simulink model "Lab2Skeleton"  (R2022a)
settings: Solver=ode1  StartTime=0.0  StopTime=70  FixedStep=0.01  RelTol=1e-3  EnableMultiTasking=on
PostLoadFcn:
  | p=1:640; % pixels from left to right
  | 
  | Obtained_angles=(320-p).*(57/640)*pi./180;  % Kinect's horizontal FOV = 57 degrees
  | 
  | S=400; % S = Size of the 2D Map matrix... the highet S is the higher resolution we would end up with - %00 might be high for Embedded computing
undefined symbols (not defined in the file): HIL, qc_get_step_size
libraries: quarc_library x4
settings Model: ExtModeTrigDuration=2  Creator=drmadill  LastModifiedBy=jonic
settings SolverCC: AlgebraicLoopSolver=TrustRegion  PositivePriorityOrder=on
settings DataIOCC: SaveOutput=off  SignalLogging=off  DSMLogging=off  SaveTime=off  ReturnWorkspaceOutputs=off
settings DebuggingCC: UnconnectedInputMsg=warning  UnconnectedOutputMsg=warning  UnconnectedLineMsg=warning  SFMachineParentedDataDiag=warning  ArithmeticOperatorsInVariantConditions=warning
settings SFSimCC: SimUseLocalCustomCode=off  CustomCodeUndefinedFunction=UseInterfaceOnly
settings RTWCC: Description=Generic Real-Time Target  RTWUseLocalCustomCode=off
settings CodeAppCC: StateflowObjectComments=on
settings ConfigComp: CovMetricSettings=dswe

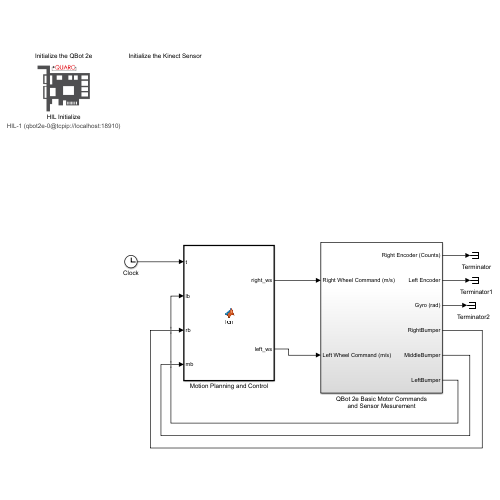
[thumbnail: Simulink's stored preview of the top-level diagram]
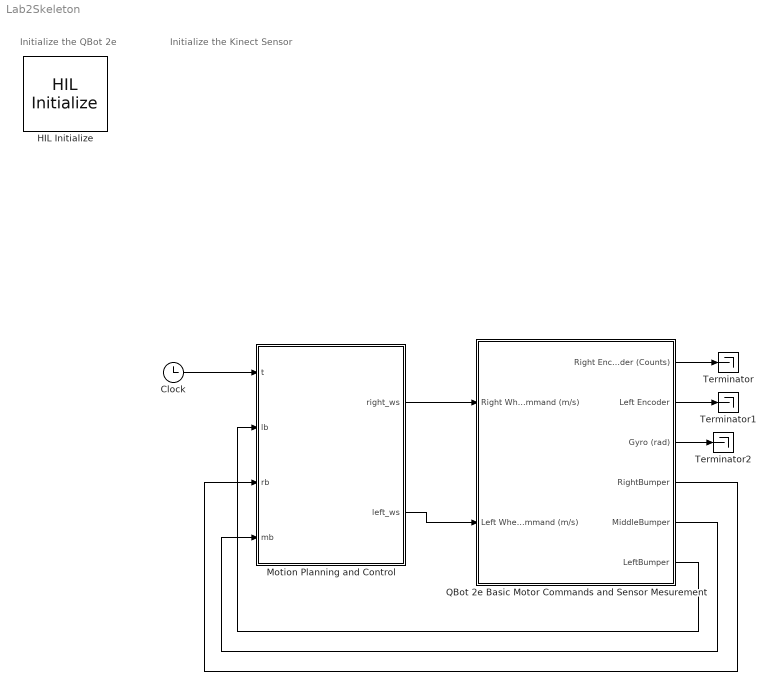
== system Lab2Skeleton ==
  note: Initialize the Kinect Sensor
  note: Initialize the QBot 2e
  Clock : Clock
  HIL Initialize : quarc_library/Data Acquisition/Generic/Configuration/HIL Initialize  Priority=-99  object_name=HIL-1  board_type=qbot2e  board_number=0@tcpip://localhost:18910  board_options=pwm0_en=1;pwm0_pin=12;pwm1_en=1;pwm1_pin=13;  exclusive=off  active=on  hardware_clocks=[]  clock_modes=[]  initial_clock_frequencies=[]  set_clock_params_at_start=off  set_clock_params_at_switch_in=off  set_clock_frequencies_at_start=off  set_clock_frequencies_at_switch_in=off  analog_input_channels=[0:5]  analog_input_configurations=[]  analog_input_maximums=[16.5 3.3 3.3 3.3 3.3 3.3]  analog_input_minimums=[0 0 0 0 0 0]  set_analog_input_params_at_start=off  set_analog_input_params_at_switch_in=off  analog_output_channels=[]  analog_output_maximums=[]  analog_output_minimums=[]  initial_analog_outputs=[]  final_analog_outputs=[]  watchdog_analog_outputs=[]  set_analog_output_params_at_start=off  set_analog_output_params_at_switch_in=off  set_analog_outputs_at_start=off  set_analog_outputs_at_switch_in=off  set_analog_outputs_at_terminate=off  set_analog_outputs_at_switch_out=off  set_analog_outputs_on_watchdog=off  digital_input_channels=[28:58]  digital_output_channels=[28:31]  digital_output_configuration=[]  initial_digital_outputs=[0]  final_digital_outputs=[0]  watchdog_digital_outputs=[]  set_digital_output_params_at_start=off  set_digital_output_params_at_switch_in=off  set_digital_outputs_at_start=on  set_digital_outputs_at_switch_in=off  set_digital_outputs_at_terminate=on  set_digital_outputs_at_switch_out=off  set_digital_outputs_on_watchdog=off  encoder_channels=[0:1]  quadrature=[4]  encoder_filter_frequency=[]  initial_encoder_counts=[0]  set_encoder_params_at_start=on  set_encoder_params_at_switch_in=off  set_encoder_counts_at_start=on  set_encoder_counts_at_switch_in=off  pwm_channels=[0:1]  pwm_modes=0  pwm_frequency=100e6 / 4095  pwm_configuration=[0]  pwm_alignment=[0]  pwm_polarity=[1]  pwm_leading_deadband=[]  pwm_trailing_deadband=[]  initial_pwm_outputs=[0]  final_pwm_outputs=[0]  watchdog_pwm_outputs=[]  set_pwm_params_at_start=on  set_pwm_params_at_switch_in=off  set_pwm_outputs_at_start=on  set_pwm_outputs_at_switch_in=off  set_pwm_outputs_at_terminate=on  set_pwm_outputs_at_switch_out=off  set_pwm_outputs_on_watchdog=off  other_output_channels=[2000:2001 14000 16000]  initial_other_outputs=[0 0 0 7]  final_other_outputs=[0 0 0 7]  watchdog_other_outputs=[]  set_other_outputs_at_start=on  set_other_outputs_at_switch_in=off  set_other_outputs_at_terminate=on  set_other_outputs_at_switch_out=off  set_other_outputs_on_watchdog=off
  Motion Planning and Control : MATLAB Function  TreatAsAtomicUnit=on  SystemSampleTime=qc_get_step_size
  QBot 2e Basic Motor Commands and Sensor Mesurement : Subsystem
  Terminator : Terminator
  Terminator1 : Terminator
  Terminator2 : Terminator
  wires:
  Clock/1 -> Motion Planning and Control/1(t)
  QBot 2e Basic Motor Commands and Sensor Mesurement/4(RightBumper) -> Motion Planning and Control/3(rb)
  QBot 2e Basic Motor Commands and Sensor Mesurement/5(MiddleBumper) -> Motion Planning and Control/4(mb)
  QBot 2e Basic Motor Commands and Sensor Mesurement/6(LeftBumper) -> Motion Planning and Control/2(lb)
  Motion Planning and Control/1(right_ws) -> QBot 2e Basic Motor Commands and Sensor Mesurement/1(Right Wheel Command (m/s))
  Motion Planning and Control/2(left_ws) -> QBot 2e Basic Motor Commands and Sensor Mesurement/2(Left Wheel Command (m/s))
  QBot 2e Basic Motor Commands and Sensor Mesurement/1(Right Encoder (Counts)) -> Terminator/1
  QBot 2e Basic Motor Commands and Sensor Mesurement/2(Left Encoder) -> Terminator1/1
  QBot 2e Basic Motor Commands and Sensor Mesurement/3(Gyro (rad)) -> Terminator2/1

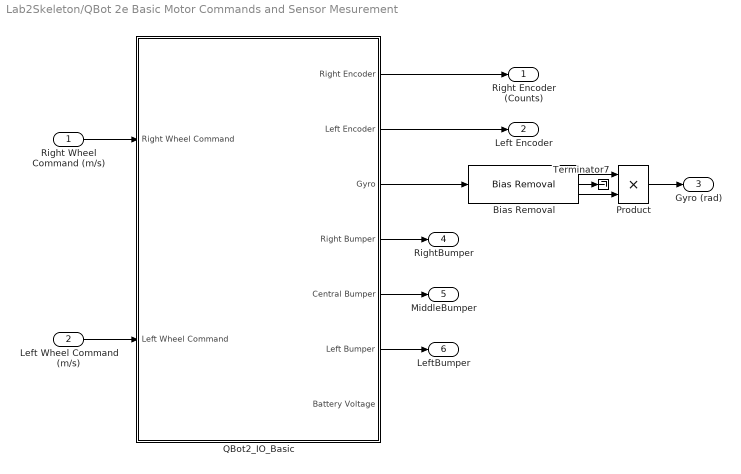
== system Lab2Skeleton/QBot 2e Basic Motor Commands and Sensor Mesurement ==
  Right Wheel Command (m/s) : Inport
  Left Wheel Command (m/s) : Inport  Port=2
  Bias Removal : quarc_library/Discrete/Bias Removal  start_time=3  end_time=4  switch_id=0  sample_time=qc_get_step_size
      settings: SourceProductName=QUARC Targets
  Product : Product  RndMeth=Zero
  QBot2_IO_Basic : Subsystem
  Terminator7 : Terminator
  Right Encoder (Counts) : Outport  VectorParamsAs1DForOutWhenUnconnected=off
  Left Encoder : Outport  Port=2  VectorParamsAs1DForOutWhenUnconnected=off
  Gyro (rad) : Outport  Port=3  VectorParamsAs1DForOutWhenUnconnected=off
  RightBumper : Outport  Port=4  VectorParamsAs1DForOutWhenUnconnected=off
  MiddleBumper : Outport  Port=5  VectorParamsAs1DForOutWhenUnconnected=off
  LeftBumper : Outport  Port=6  VectorParamsAs1DForOutWhenUnconnected=off
  wires:
  Right Wheel Command (m/s)/1 -> QBot2_IO_Basic/1(Right Wheel Command)
  Left Wheel Command (m/s)/1 -> QBot2_IO_Basic/2(Left Wheel Command)
  QBot2_IO_Basic/1(Right Encoder) -> Right Encoder (Counts)/1
  QBot2_IO_Basic/2(Left Encoder) -> Left Encoder/1
  Bias Removal/2 -> Terminator7/1
  Bias Removal/1 -> Product/1
  Bias Removal/3 -> Product/2
  Product/1 -> Gyro (rad)/1
  QBot2_IO_Basic/3(Gyro) -> Bias Removal/1
  QBot2_IO_Basic/4(Right Bumper) -> RightBumper/1
  QBot2_IO_Basic/6(Left Bumper) -> LeftBumper/1
  QBot2_IO_Basic/5(Central Bumper) -> MiddleBumper/1

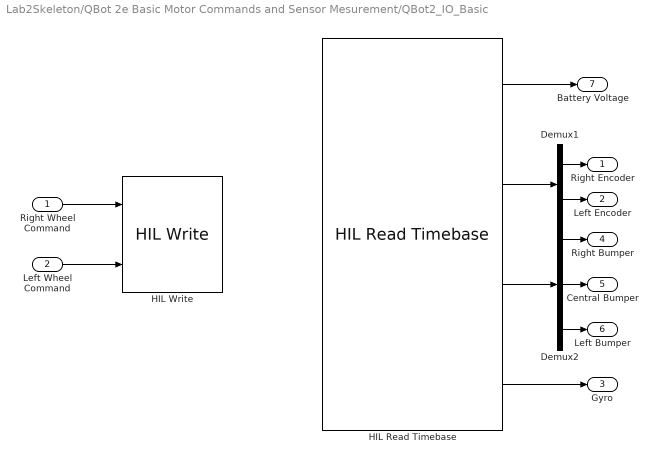
== system Lab2Skeleton/QBot 2e Basic Motor Commands and Sensor Mesurement/QBot2_IO_Basic ==
  Right Wheel Command : Inport
  Left Wheel Command : Inport  Port=2
  Demux1 : Demux  Outputs=2
  Demux2 : Demux  Outputs=3
  HIL Read Timebase : quarc_library/Data Acquisition/Generic/Timebases/HIL Read Timebase  object_name=HIL-1  clock=0  analog_channels=0  encoder_channels=0:1  digital_channels=28:30  other_channels=1002  active=on  vector_output=on  data_type_mode=Inherit via back propagation  encoder_data_type=double  digital_data_type=boolean  overflow_mode=Synchronize (for simulated cards only)  samples_in_buffer=1+0*max(ceil(1/qc_get_step_size), 1)
  HIL Write : quarc_library/Data Acquisition/Generic/Immediate I//O/HIL Write  object_name=HIL-1  analog_channels=[]  pwm_channels=[]  digital_channels=[]  other_channels=[2000:2001]  sample_time=-1  active=on  vector_input=off
  Right Encoder : Outport  VectorParamsAs1DForOutWhenUnconnected=off
  Left Encoder : Outport  Port=2  VectorParamsAs1DForOutWhenUnconnected=off
  Gyro : Outport  Port=3  VectorParamsAs1DForOutWhenUnconnected=off
  Right Bumper : Outport  Port=4  VectorParamsAs1DForOutWhenUnconnected=off
  Central Bumper : Outport  Port=5  VectorParamsAs1DForOutWhenUnconnected=off
  Left Bumper : Outport  Port=6  VectorParamsAs1DForOutWhenUnconnected=off
  Battery Voltage : Outport  Port=7  VectorParamsAs1DForOutWhenUnconnected=off
  wires:
  HIL Read Timebase/1 -> Battery Voltage/1
  HIL Read Timebase/3 -> Demux2/1
  HIL Read Timebase/4 -> Gyro/1
  Demux1/1 -> Right Encoder/1
  Demux1/2 -> Left Encoder/1
  Right Wheel Command/1 -> HIL Write/1
  Left Wheel Command/1 -> HIL Write/2
  HIL Read Timebase/2 -> Demux1/1
  Demux2/1 -> Right Bumper/1
  Demux2/2 -> Central Bumper/1
  Demux2/3 -> Left Bumper/1

== matlab function Lab2Skeleton/Motion Planning and Control ==
  settings: sampleTime=qc_get_step_size
  data: right_ws output; t input; lb input; rb input; left_ws output; mb input
function [right_ws, left_ws] = fcn(t, lb, rb, mb)
    %#codegen
    
    persistent flag_rotate
    persistent flag_move
    persistent flag_rotate_back
    persistent flag_move_back
    
    if isempty(flag_rotate) flag_rotate=0; end
    if isempty(flag_move) flag_move=0; end
    if isempty(flag_rotate_back) flag_rotate_back=0; end
    if isempty(flag_move_back) flag_move_back=0; end
    
    % For ease of not metting up other movements, I decided to make the 
    % movement time for each step a variable. Thsi should allow us to
    % change the time for rotation without messing up the times for forward
    % movement since they are summed together instead of hardcoded
    
    t_m1 = 4; % move 4s at 0.25 m/s for 1m movement
    t_m2 = 2; % TODO: BAILEY WHAT SHOULD THIS t BE????
    t_m3 = 4; % move 4s at 0.25 m/s for 1m movement
    t_m4 = 2; % TODO: BAILEY WHAT SHOULD THIS t BE????
    t_m5 = 8; % move 8s at 0.25 m/s for 2m movement
    
    if t < t_m1 % Move forward 1m
        left_ws = 0.25;
        right_ws = 0.25;
    
    elseif t < (t_m1 + t_m2) % Move with a 1m radius of rotation for 90 degrees
        R_turn = 1; % m
        v_base = 0.4; % m/s; velocity of chassis
        v_d = rotate(R_turn, v_base);
        left_ws = v_base - v_d;
        right_ws = v_base + v_d;
    
    elseif t < (t_m1 + t_m2 + t_m3) % Move forward 1m
        left_ws = 0.25;
        right_ws = 0.25;
    
    elseif t < (t_m1 + t_m2 + t_m3 + t_m4) % Move with a 0.5m radius of rotation for 90 degrees
        R_turn = 0.5; % m
        v_base = 0.3; % m/s; velocity of chassis
        v_d = rotate(R_turn, v_base);

        % Switch the signs for the v_d parameter to rotate in the opposite 
        % direction
        left_ws = v_base + v_d;
        right_ws = v_base - v_d;
    
    elseif t < (t_m1 + t_m2 + t_m3 + t_m4 + t_m5) % Move forward 2m
        left_ws = 0.25;
        right_ws = 0.25;

    else
        left_ws = 0;
        right_ws = 0;
    end
end


%%%%%%%%%%%%%%%%%%%%%%%%%%%%%%%%%%%%%%%%%%%%%%%%%%%%%%%%%%%%%%%%%%%%%%%%%%%
%                                                                         %
% Function to rotate the robot about some radius, R_turn, at some         %
% tangential velocity of the chassis, v_base.                             %
%                                                                         %
%%%%%%%%%%%%%%%%%%%%%%%%%%%%%%%%%%%%%%%%%%%%%%%%%%%%%%%%%%%%%%%%%%%%%%%%%%%
function [v_d] = rotate(R_turn, v_base)
    wheel_sep = 0.235; % The distance between the robot wheels
    v_d = - (wheel_sep/2) * (v_base/R_turn); % The differential velocity between the wheels
end
